simulink model "Model13"  (R2020a)
settings: Solver=ode15s  StartTime=0.0  StopTime=71  RelTol=1e-3
undefined symbols (not defined in the file): a, a0, a1, a10, a11, a12, a13, a14, a15, a16, a17, a2, a3, a4, a5, a6, a7, a8, a9, alpha, Area, b, b1, b11, b12, b2, banking_indy, bankingON, C_fuel, camber, curveCenters, Cx, Cz, distanceThreshold, g, init_x_pos, init_y_pos, init_yaw, IT, K_wear, l_f, l_r, longStraight, m_fuel, mT, overlapThreshold, radius_second_lane, rho_0, rho_1, shortStraight, slipstreamON, trajec, turn, TyreContactAreaFront, TyreContactAreaRear, w1, w2
libraries: simulink x5, cstblocks x1
(part 2 of 2)

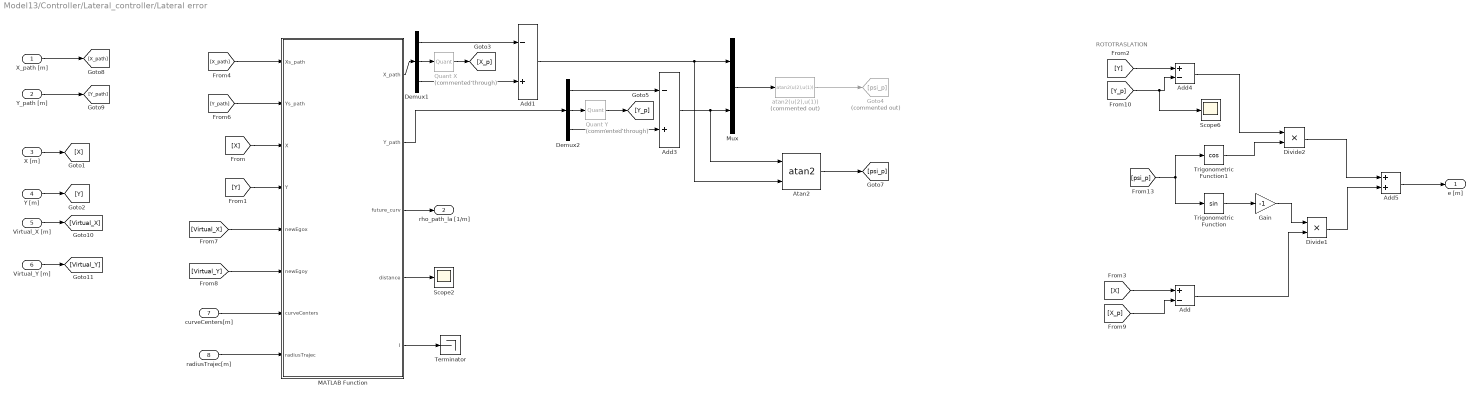
== system Model13/Controller/Lateral_controller/Lateral error ==
  note: ROTOTRASLATION
  X_path [m] : Inport
  Y_path [m] : Inport  Port=2
  X [m] : Inport  Port=3
  Y [m] : Inport  Port=4
  Virtual_X [m] : Inport  Port=5
  Virtual_Y [m] : Inport  Port=6
  curveCenters[m] : Inport  Port=7  Unit=m
  radiusTrajec[m] : Inport  Port=8  Unit=m
  Add : Sum  Inputs=+-
  Add1 : Sum  Inputs=-+
  Add3 : Sum  Inputs=-+
  Add4 : Sum  Inputs=+-
  Add5 : Sum
  Atan2 : Trigonometry  Operator=atan2
  Demux1 : Demux  Outputs=3
  Demux2 : Demux  Outputs=3
  Divide1 : Product  Inputs=**
  Divide2 : Product  Inputs=**
  Gain : Gain  Gain=-1
  Goto4 : Goto  Commented=on  GotoTag=psi_p
  MATLAB Function : MATLAB Function  TreatAsAtomicUnit=on
  Mux : Mux  Inputs=2
  Quant X : Quantizer  Commented=through  QuantizationInterval=0.007
  Quant Y : Quantizer  Commented=through  QuantizationInterval=0.01
  Scope2 : Scope
  Scope6 : Scope
  Terminator : Terminator
  Trigonometric Function : Trigonometry
  Trigonometric Function1 : Trigonometry  Operator=cos
  atan2(u(2),u(1)) : Fcn  Commented=on  Expr=atan2(u(2),u(1))
  e [m] : Outport  VectorParamsAs1DForOutWhenUnconnected=off
  rho_path_la [1/m] : Outport  Port=2  VectorParamsAs1DForOutWhenUnconnected=off
  wires:
  Demux1/2 -> Quant X/1
  Demux1/3 -> Add1/2
  Add3/1 -> Atan2/1, Mux/2
  Demux2/2 -> Quant Y/1
  MATLAB Function/2(Y_path) -> Demux2/1
  Demux2/1 -> Add3/1
  Demux2/3 -> Add3/2
  MATLAB Function/4(distance) -> Scope2/1
  MATLAB Function/1(X_path) -> Demux1/1
  Trigonometric Function1/1 -> Divide2/2
  Demux1/1 -> Add1/1
  [Y_p] -> Scope6/1, Add4/2
  Divide1/1 -> Add5/2
  Divide2/1 -> Add5/1
  [X_p] -> Add/2
  [psi_p] -> Trigonometric Function1/1, Trigonometric Function/1
  Trigonometric Function/1 -> Gain/1
  Add1/1 -> Atan2/2, Mux/1
  Add/1 -> Divide1/2
  Add4/1 -> Divide2/1
  Gain/1 -> Divide1/1
  X_path [m]/1 -> [X_path]
  Y_path [m]/1 -> [Y_path]
  X [m]/1 -> [X]
  Y [m]/1 -> [Y]
  [X] -> MATLAB Function/3(X)
  [Y] -> MATLAB Function/4(Y)
  [Y] -> Add4/1
  [X] -> Add/1
  Quant X/1 -> [X_p]
  Quant Y/1 -> [Y_p]
  atan2(u(2),u(1))/1 -> Goto4/1
  MATLAB Function/3(future_curv) -> rho_path_la [1/m]/1
  Mux/1 -> atan2(u(2),u(1))/1
  Atan2/1 -> [psi_p]
  Add5/1 -> e [m]/1
  [X_path] -> MATLAB Function/1(Xs_path)
  [Y_path] -> MATLAB Function/2(Ys_path)
  Virtual_X [m]/1 -> [Virtual_X]
  Virtual_Y [m]/1 -> [Virtual_Y]
  [Virtual_X] -> MATLAB Function/5(newEgox)
  [Virtual_Y] -> MATLAB Function/6(newEgoy)
  curveCenters[m]/1 -> MATLAB Function/7(curveCenters)
  radiusTrajec[m]/1 -> MATLAB Function/8(radiusTrajec)
  MATLAB Function/5(I) -> Terminator/1

== matlab function Model13/Controller/Lateral_controller/Lateral error/MATLAB Function ==
  data: Xs_path input; Ys_path input; X_path output; X input; Y input; newEgox input; newEgoy input; curveCenters input; radiusTrajec input; Y_path output; future_curv output; distance output; I output
function [X_path,Y_path,future_curv,distance,I] = fcn(Xs_path,Ys_path,X,Y, newEgox, newEgoy, curveCenters, radiusTrajec)
% ...
% returns coordinates, heading and distance of the nearest path point
% do not consider the car going backwards 

Xs_path_tmp=Xs_path(:);
Ys_path_tmp=Ys_path(:);

[distance,Itmp]=min(sqrt((Xs_path_tmp-X).^2+(Ys_path_tmp-Y).^2));

I=Itmp;

if I == 1
    X_path=[Xs_path(length(Xs_path)), Xs_path(I), Xs_path(I+1)]';
    Y_path=[Ys_path(length(Xs_path)), Xs_path(I), Xs_path(I+1)]';
elseif I == length(Xs_path)
    X_path=[Xs_path(I-1), Xs_path(I), Xs_path(1)]';
    Y_path=[Ys_path(I-1), Xs_path(I), Xs_path(1)]';
else
    X_path=Xs_path(I-1:I+1);
    Y_path=Ys_path(I-1:I+1);
end

% takes the future curvature
% long straight 1
if newEgoy < curveCenters(1,2) && newEgox >= curveCenters(4,1) && newEgox <= curveCenters(1,1)
    future_curv = 0;
% long straight 2
elseif newEgoy > curveCenters(2,2) && newEgox >= curveCenters(4,1) && newEgox <= curveCenters(1,1)
    future_curv = 0;
% short straigt 1
elseif newEgox > 0 && newEgoy >= curveCenters(1,2) && newEgoy <= curveCenters(2,2)
    future_curv = 0;
% short straigt 2
elseif newEgox < 0 && newEgoy >= curveCenters(1,2) && newEgoy <= curveCenters(2,2)
    future_curv = 0;
% curve 1
elseif newEgox > curveCenters(1,1) && newEgoy < curveCenters(1,2)
    future_curv = 1/radiusTrajec;
% curve 2
elseif newEgox > curveCenters(2,1) && newEgoy > curveCenters(2,2)
    future_curv = 1/radiusTrajec;
% curve 3
elseif newEgox < curveCenters(3,1) && newEgoy > curveCenters(3,2)
    future_curv = 1/radiusTrajec;
% curve 4
elseif newEgox < curveCenters(4,1) && newEgoy < curveCenters(4,2)
    future_curv = 1/radiusTrajec;
% default else
else
    future_curv = 0;
end

== matlab function Model13/Controller/Longitudinal_controller/v_ref ==
  data: egox input; egoy input; trajec input; ref output
function ref = vel_ref(egox, egoy, trajec)

% index = floor(mod(pos*10, max_pos) + 1);
% thresh1 = 60;
% thresh2 = 20;
% from = max(1, index - thresh1);
% to = min(max_pos, index + thresh2);
% 
% real_index = from;
% min_dist = pdist2([trajec(2,real_index),trajec(3,real_index)],[egox, egoy]);
% for i=from+1:to
%     new_dist = pdist2([trajec(2,i),trajec(3,i)],[egox, egoy]);
%     if new_dist < min_dist
%         min_dist = new_dist;
%         real_index = i;
%     end
% end
distArray = (egox - trajec(2,:)).^2 + (egoy - trajec(3,:)).^2;
[~, real_index] = min(distArray);
ref = trajec(5, real_index);

% function ref = vel_ref(egox, egoy, trajec, cur_vel)
% 
% thresh = 5;
% maxp = 10;
% index = find( (abs(trajec(2,:) - egox) < thresh) & (abs(trajec(3,:) - egoy) < thresh), maxp);
% 
% if (isempty(index))
%     ref = cur_vel;
% else
%     
%     size_index = size(index, 2);
% 
%     real_index = index(1,1);
%     min_dist = pdist2([trajec(2,real_index),trajec(3,real_index)],[egox, egoy]);
% 
%     for i=2:size_index
%         new_dist = pdist2([trajec(2,index(1,i)),trajec(3,index(1,i))],[egox, egoy]);
%         if new_dist < min_dist
%             min_dist = new_dist;
%             real_index = index(1,i);
%         end
%     end
%     
%     ref = trajec(5, real_index);
% end

== matlab function Model13/DynamicModel/Banking ==
  data: x input; res output; y input; curveCenters input; longStraight input; shortStraight input; curve input; bankingON input; banking_indy input
function res = calculateBanking(x, y, curveCenters, ...
    longStraight, shortStraight, curve, ...
    bankingON, banking_indy)

% coder.extrinsic('evalin')
% coder.extrinsic('fitresult')
% fun = evalin('base','fitresult');

init_x = -271.4;
totL = 4023.4;
initD = pdist2([init_x, 0], [curveCenters(1,1),0]);

R = curve * 2 / pi;


if (bankingON < 1)
    res = 0;
else
    % long straight 1
    if y < curveCenters(1,2) && x >= curveCenters(4,1) && x <= curveCenters(1,1)
        d = pdist2([x, 0],[init_x, 0]);
        l = (totL - d)*(x < init_x) + ...
            (d)*(x >= init_x);
    % long straight 2
    elseif y > curveCenters(2,2) && x >= curveCenters(4,1) && x <= curveCenters(1,1)
        d = pdist2([x, 0],[curveCenters(2,1),0]);
        l = d + initD + shortStraight + 2*curve;
    % short straigt 1
    elseif x > 0 && y >= curveCenters(1,2) && y <= curveCenters(2,2)
        d = pdist2([y, 0],[curveCenters(1,2),0]);
        l = d + initD + curve;
    % short straigt 2
    elseif x < 0 && y >= curveCenters(1,2) && y <= curveCenters(2,2)
        d = pdist2([y, 0],[curveCenters(3,2),0]);
        l = d + initD + longStraight + shortStraight + 3*curve;
    % curve 1
    elseif x > curveCenters(1,1) && y < curveCenters(1,2)
        ang = asin((x - curveCenters(1,1))/pdist2([x,y],curveCenters(1,:)));
        l = ang * R + initD;
    % curve 2
    elseif x > curveCenters(2,1) && y > curveCenters(2,2)
        ang = asin((y - curveCenters(2,2))/pdist2([x,y],curveCenters(2,:)));
        l = ang * R + initD + curve + shortStraight;
    % curve 3
    elseif x < curveCenters(3,1) && y > curveCenters(3,2)
        ang = asin((-x + curveCenters(3,1))/pdist2([x,y],curveCenters(3,:)));
        l = ang * R + initD + curve*2 + shortStraight + longStraight;
    % curve 4
    elseif x < curveCenters(4,1) && y < curveCenters(4,2)
        ang = asin((-y + curveCenters(4,2))/pdist2([x,y],curveCenters(4,:)));
        l = ang * R + initD + curve*3 + shortStraight*2 + longStraight;
    % default else
    else 
        l = 0;
    end
    
    %res = fun(l);
    res = banking_indy(ceil(l*10),1);
    %res = 0;
end

% function res = calculateBanking(x, y, curveCenters, ...
%     bankingThresholdLong, bankingThresholdShort, bankingAngle, midY, ...
%     bankingON)
% if (bankingON < 1)
%     res = 0;
% else
%     if(y < curveCenters(1,2) || y > curveCenters(2,2)) 
%        if(abs(x) < curveCenters(1,1) - bankingThresholdLong)
%            res = 0;
%        elseif (abs(x) > curveCenters(1,1))
%            res = bankingAngle;
%        else
%            res = bankingAngle*( 1 - ((abs(x) -  curveCenters(1,1))/(-bankingThresholdLong)) );
%        end
%     else
%         if (abs(y-midY) < curveCenters(2,2) - bankingThresholdShort - midY)
%             res = 0;
%         else
%             res = bankingAngle*( 1 - ((abs(y-midY) -  curveCenters(2,2) + midY)/(-bankingThresholdShort)) );
%         end
%     end
% end

== matlab function Model13/Controller/Lateral_controller/periodic ==
  data: yaw input; periodicYaw output
function periodicYaw = periodic(yaw)

periodicYaw = abs(yaw) - (2*pi * floor(abs(yaw)/(2*pi)));

== matlab function Model13/DynamicModel/WindEffect ==
  data: rho_0 input; aerodynamic_coeff output; rho_1 input; ego_x input; ego_y input; opp_x input; opp_y input; distanceThreshold input; overlapThreshold input; alpha input; curveCenters input; slipstreamON input
function aerodynamic_coeff = windEffect(rho_0, rho_1, ego_x, ego_y, ... 
    opp_x, opp_y, distanceThreshold, overlapThreshold, alpha, curveCenters, ...
    slipstreamON)

if(slipstreamON < 1)
    aerodynamic_coeff = rho_0;
else
    %give in output rho_0 if too distant from other vehicle
    %rho_1 otherwise
    distanceThresholdCurve =  alpha * distanceThreshold;
    overlapThresholdCurve =  alpha * overlapThreshold;

    if  ego_x > curveCenters(1,1) && ego_y < curveCenters(1,2) %check if in the first curve
        ego_radius = sqrt((ego_x - curveCenters(1,1))^2 + (ego_y - curveCenters(1,2))^2);
        opp_radius = sqrt((opp_x - curveCenters(1,1))^2 + (opp_y - curveCenters(1,2))^2);
        if abs(ego_radius - opp_radius) < overlapThresholdCurve && ...
                sqrt((ego_x - opp_x)^2 + (ego_y - opp_y)^2) < distanceThresholdCurve && ...
                ego_y < opp_y
            aerodynamic_coeff = rho_1;
        else
           aerodynamic_coeff = rho_0;
        end
    elseif ego_x > curveCenters(2,1) && ego_y > curveCenters(2,2) %check if in the second curve
        ego_radius = sqrt((ego_x - curveCenters(2,1))^2 + (ego_y - curveCenters(2,2))^2);
        opp_radius = sqrt((opp_x - curveCenters(2,1))^2 + (opp_y - curveCenters(2,2))^2);
        if abs(ego_radius - opp_radius) < overlapThresholdCurve && ...
                sqrt((ego_x - opp_x)^2 + (ego_y - opp_y)^2) < distanceThresholdCurve && ...
                ego_x > opp_x
            aerodynamic_coeff = rho_1;
        else
           aerodynamic_coeff = rho_0;
        end
    elseif ego_x < curveCenters(3,1) && ego_y > curveCenters(3,2) %check if in the third curve
        ego_radius = sqrt((ego_x - curveCenters(3,1))^2 + (ego_y - curveCenters(3,2))^2);
        opp_radius = sqrt((opp_x - curveCenters(3,1))^2 + (opp_y - curveCenters(3,2))^2);
        if abs(ego_radius - opp_radius) < overlapThresholdCurve && ...
                sqrt((ego_x - opp_x)^2 + (ego_y - opp_y)^2) < distanceThresholdCurve && ...
                ego_y > opp_y
            aerodynamic_coeff = rho_1;
        else
           aerodynamic_coeff = rho_0;
        end
    elseif ego_x < curveCenters(4,1) && ego_y < curveCenters(4,2) %check if in the fourth curve
        ego_radius = sqrt((ego_x - curveCenters(4,1))^2 + (ego_y - curveCenters(4,2))^2);
        opp_radius = sqrt((opp_x - curveCenters(4,1))^2 + (opp_y - curveCenters(4,2))^2);
        if abs(ego_radius - opp_radius) < overlapThresholdCurve && ...
                sqrt((ego_x - opp_x)^2 + (ego_y - opp_y)^2) < distanceThresholdCurve && ...
                ego_x < opp_x
            aerodynamic_coeff = rho_1;
        else
           aerodynamic_coeff = rho_0;
        end
    else
        %check for which straights
        if ego_y < curveCenters(1,2) && ego_x >= curveCenters(4,1) && ego_x <= curveCenters(1,1)
           %first long straight
           if abs(ego_y - opp_y) < overlapThreshold && ...
                   abs(opp_x - ego_x) < distanceThreshold && ...
                   ego_x < opp_x
               aerodynamic_coeff = rho_1;
           else
               aerodynamic_coeff = rho_0;
           end

        elseif ego_y > curveCenters(2,2) && ego_x >= curveCenters(3,1) && ego_x <= curveCenters(2,1)
           %second long straight
           if abs(ego_y - opp_y) < overlapThreshold && ...
                   abs(opp_x - ego_x) < distanceThreshold && ...
                   ego_x > opp_x
               aerodynamic_coeff = rho_1;
           else
               aerodynamic_coeff = rho_0;
           end

        elseif ego_x > curveCenters(1,1) && ego_y >= curveCenters(1,2) && ego_y <= curveCenters(2,2)
           %first short straight
           if abs(ego_x - opp_x) < overlapThreshold && ...
                   abs(opp_y - ego_y) < distanceThreshold && ...
                   ego_y < opp_y
               aerodynamic_coeff = rho_1;
           else
               aerodynamic_coeff = rho_0;
           end

        elseif ego_x < curveCenters(3,1) && ego_y >= curveCenters(4,2) && ego_y <= curveCenters(3,2)
           %second short straight
           if abs(ego_x - opp_x) < overlapThreshold && ...
                   abs(opp_y - ego_y) < distanceThreshold && ...
                   ego_y > opp_y
               aerodynamic_coeff = rho_1;
           else
               aerodynamic_coeff = rho_0;
           end

        else
            aerodynamic_coeff = rho_0;
        end
    end
end

== matlab function Model13/Controller/Lateral_controller/lateral error ==
  data: egox input; egoy input; trajec input; error output; future_curv output; cur_yaw input; lookAhead input; curveCenters input; radiusTrajec input
function [error,future_curv] = lateral_error(egox, egoy, trajec, cur_yaw, lookAhead, curveCenters, radiusTrajec)

newEgox = egox + lookAhead*cos(cur_yaw);
newEgoy = egoy + lookAhead*sin(cur_yaw);

distArray = (egox - trajec(2,:)).^2 + (egoy - trajec(3,:)).^2;
[min_dist, real_index] = min(distArray);

min_dist = sqrt(min_dist);

v1 = [newEgox - egox, newEgoy - egoy, 0];
v2 = [trajec(2, real_index) - egox, trajec(3, real_index) - egoy, 0];
C = cross(v1, v2);
if sign(C(3)) == 1
    error = -min_dist;
elseif sign(C(3)) == -1
    error = min_dist;
else
    error = 0;
end

% long straight 1
if newEgoy < curveCenters(1,2) && newEgox >= curveCenters(4,1) && newEgox <= curveCenters(1,1)
    future_curv = 0;
% long straight 2
elseif newEgoy > curveCenters(2,2) && newEgox >= curveCenters(4,1) && newEgox <= curveCenters(1,1)
    future_curv = 0;
% short straigt 1
elseif newEgox > 0 && newEgoy >= curveCenters(1,2) && newEgoy <= curveCenters(2,2)
    future_curv = 0;
% short straigt 2
elseif newEgox < 0 && newEgoy >= curveCenters(1,2) && newEgoy <= curveCenters(2,2)
    future_curv = 0;
% curve 1
elseif newEgox > curveCenters(1,1) && newEgoy < curveCenters(1,2)
    future_curv = 1/radiusTrajec;
% curve 2
elseif newEgox > curveCenters(2,1) && newEgoy > curveCenters(2,2)
    future_curv = 1/radiusTrajec;
% curve 3
elseif newEgox < curveCenters(3,1) && newEgoy > curveCenters(3,2)
    future_curv = 1/radiusTrajec;
% curve 4
elseif newEgox < curveCenters(4,1) && newEgoy < curveCenters(4,2)
    future_curv = 1/radiusTrajec;
% default else
else
    future_curv = 0;
end
